simulink model "AB1"  (R2017a)
settings: Solver=VariableStepAuto  StartTime=0.0  StopTime=10.0  RelTol=1e-3
values from neighbouring files (symbols this model uses):
  k = 7    [AB1.m]
undefined symbols (not defined in the file or in its folder): A, B, C
settings Model: Creator=mariajulia  LastModifiedBy=mariajulia

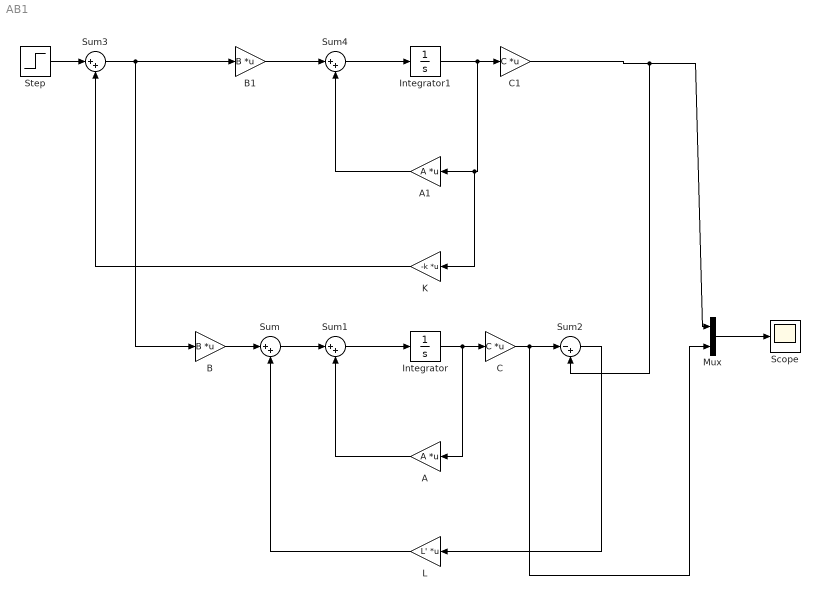
== system AB1 ==
  A : Gain  Gain=A  Multiplication=Matrix(K*u)
  A1 : Gain  Gain=A  Multiplication=Matrix(K*u)
  B : Gain  Gain=B  Multiplication=Matrix(K*u)
  B1 : Gain  Gain=B  Multiplication=Matrix(K*u)
  C : Gain  Gain=C  Multiplication=Matrix(K*u)
  C1 : Gain  Gain=C  Multiplication=Matrix(K*u)
  Integrator : Integrator
  Integrator1 : Integrator
  K : Gain  Gain=-k  Multiplication=Matrix(K*u)
  L : Gain  Gain=L'  Multiplication=Matrix(K*u)
  Mux : Mux  Inputs=2
  Scope : Scope
  Step : Step  SampleTime=0
  Sum{,1,3..4} (4 alike) : Sum  Inputs=|++
  Sum2 : Sum  Inputs=|-+
  wires:
  Mux/1 -> Scope/1
  Integrator/1 -> C/1, A/1
  Sum1/1 -> Integrator/1
  A/1 -> Sum1/2
  L/1 -> Sum/2
  Sum2/1 -> L/1
  C/1 -> Mux/2, Sum2/1
  B/1 -> Sum/1
  Sum/1 -> Sum1/1
  A1/1 -> Sum4/2
  Sum4/1 -> Integrator1/1
  C1/1 -> Mux/1, Sum2/2
  Sum3/1 -> B/1, B1/1
  B1/1 -> Sum4/1
  K/1 -> Sum3/2
  Integrator1/1 -> K/1, A1/1, C1/1
  Step/1 -> Sum3/1
